simulink model "DDCU_wxt_v02"  (R2014a)
settings: Solver=ode45  StartTime=0.0  StopTime=50  FixedStep=0.0005  RelTol=1e-3
values from neighbouring files (symbols this model uses):
  ag_thr = 0.4*g    (= 3.924)    [Veh_Par_wxt.m]
  B = 2.25    [Veh_Par_wxt.m]
  bra_pre_em = 12    [Veh_Par_wxt.m]
  bra_pre_gz2 = 12/3    (= 4)    [Veh_Par_wxt.m]
  bra_pre_gz34 = 12/3    (= 4)    [Veh_Par_wxt.m]
  bra_pre_yd = 12/2    (= 6)    [Veh_Par_wxt.m]
  brakepre_dem_data = [0 1 2 3 4 5 6 7 8 9 10 11 12]    [Veh_Par_wxt.m]
  brakeTrq_dem_data = [0 218.198 436.396 654.594 872.792 1090.99 1309.188 1527.386 1745.584 1963.782 2181.98 2400.178 2618.376]    [Veh_Par_wxt.m]
  bratrq_max = 4*2618.376    (= 10473.504)    [Veh_Par_wxt.m]
  eff_tran = 0.75    [Veh_Par_wxt.m]
  G = Mass*g    (= 36297)    [Veh_Par_wxt.m]
  kd1 = 1    [Veh_Par_wxt.m]
  kd2 = 1    [Veh_Par_wxt.m]
  kd3 = 1    [Veh_Par_wxt.m]
  ki1 = 1    [Veh_Par_wxt.m]
  ki2 = 1    [Veh_Par_wxt.m]
  ki3 = 1    [Veh_Par_wxt.m]
  kp1 = 1    [Veh_Par_wxt.m]
  kp2 = 1    [Veh_Par_wxt.m]
  kp3 = 1    [Veh_Par_wxt.m]
  L = 3.12    [Veh_Par_wxt.m]
  Radius = 0.20    (= 0.2)    [Veh_Par_wxt.m]
  s_opt_yi_add = 0.05    [Veh_Par_wxt.m]
  s_opt_zhuan_add = 0.05    [Veh_Par_wxt.m]
  spd_map_mot = [0 100 200 300 360 400 500 600 700 800 900]*tras_ratio    [Veh_Par_wxt.m]
  speed_thr_park = 5/3.6/Radius*30/pi    (= 66.3145596216)    [Veh_Par_wxt.m]
  trq_map_mot = [1200 1200 1200 1200 1200 1080 864 720 617 540 480]/tras_ratio    [Veh_Par_wxt.m]
  v_thr1_b = 5    [Veh_Par_wxt.m]
  v_thr2_b = 20    [Veh_Par_wxt.m]
  v_thr_park = 5    [Veh_Par_wxt.m]
undefined symbols (not defined in the file or in its folder): DiscIntNeverNeededParam
libraries: simulink x17, Solver_SF x1
(part 1 of 5)
settings Model: Creator=wxt  LastModifiedBy=wxt

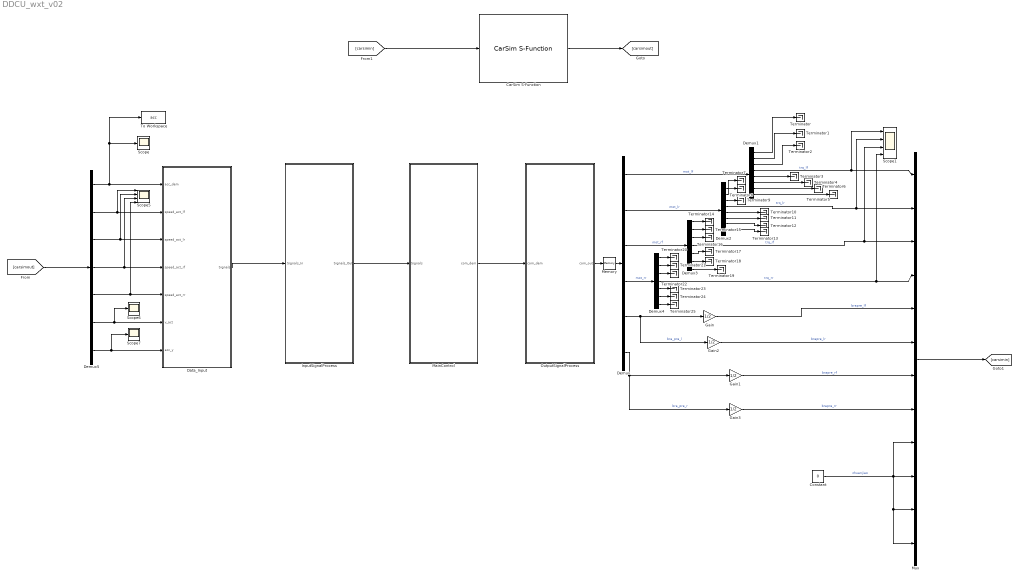
== system DDCU_wxt_v02 ==
  CarSim S-Function : Solver_SF/CarSim S-Function  Priority=1  VehicleCode=i_i  SIMFILE=lqddcuv01
  Constant : Constant  Value=0
  Data_Input : Subsystem
  Demux : Demux  Outputs=6
  Demux1 : Demux  Outputs=8
  Demux2 : Demux  Outputs=8
  Demux3 : Demux  Outputs=7
  Demux4 : Demux  Outputs=7
  Demux5 : Demux  Outputs=7
  Gain{,1..3} (4 alike) : Gain  Gain=1/2
  InputSignalProcess : Subsystem
  MainControl : Subsystem
  Memory : Memory
  Mux : Mux  Inputs=12
  OutputSignalProcess : Subsystem
  Scope : Scope
  Scope1 : Scope  NumInputPorts=4
      settings: YMin=-5~-5~-5~-5  YMax=5~5~5~5
  Scope5 : Scope  NumInputPorts=4
      settings: YMin=-5~-5~-5~-5  YMax=5~5~5~5  SaveName=ScopeData5
  Scope6 : Scope
      settings: SaveName=ScopeData6
  Scope7 : Scope
      settings: SaveName=ScopeData7
  Terminator{,1..25} (26 alike) : Terminator
  To Workspace : ToWorkspace  VariableName=acc  SampleTime=-1
  wires:
  Data_Input/1(Signals) -> InputSignalProcess/1(Signals_In)
  InputSignalProcess/1(Signals_Out) -> MainControl/1(Signals)
  MainControl/1(com_dem) -> OutputSignalProcess/1(com_dem)
  OutputSignalProcess/1(com_out) -> Memory/1
  Demux/1 -> Demux1/1  "mot_lf"
  Demux/2 -> Demux2/1  "mot_lr"
  Demux/3 -> Demux3/1  "mot_rf"
  Demux/4 -> Demux4/1  "mot_rr"
  Demux/5 -> Gain2/1, Gain/1  "bra_pre_l"
  Demux/6 -> Gain3/1, Gain1/1  "bra_pre_r"
  Demux1/4 -> Mux/1, Scope1/1  "trq_lf"
  Demux2/4 -> Mux/2, Scope1/2  "trq_lr"
  Demux3/4 -> Mux/3, Scope1/3  "trq_rf"
  Demux4/4 -> Mux/4, Scope1/4  "trq_rr"
  Gain/1 -> Mux/5  "brapre_lf"
  Gain1/1 -> Mux/7  "brapre_rf"
  Gain2/1 -> Mux/6  "brapre_lr"
  Gain3/1 -> Mux/8  "brapre_rr"
  Constant/1 -> Mux/9, Mux/10, Mux/12, Mux/11  "zhuanjiao"
  CarSim S-Function/1 -> [carsimout]
  [carsimout] -> Demux5/1
  Demux5/1 -> Data_Input/1(acc_dem), To Workspace/1, Scope/1
  Demux5/2 -> Scope5/1, Data_Input/2(speed_act_lf)
  Demux5/3 -> Data_Input/3(speed_act_lr), Scope5/2
  Demux5/4 -> Data_Input/4(speed_act_rf), Scope5/3
  Demux5/5 -> Data_Input/5(speed_act_rr), Scope5/4
  Demux5/6 -> Scope6/1, Data_Input/6(v_act)
  [carsimin] -> CarSim S-Function/1
  Mux/1 -> [carsimin]
  Demux5/7 -> Scope7/1, Data_Input/7(acc_y)
  Demux1/1 -> Terminator/1
  Demux1/2 -> Terminator1/1
  Demux1/3 -> Terminator2/1
  Demux1/5 -> Terminator3/1
  Demux1/6 -> Terminator4/1
  Demux1/7 -> Terminator5/1
  Demux1/8 -> Terminator6/1
  Demux2/3 -> Terminator9/1
  Demux2/2 -> Terminator8/1
  Demux2/1 -> Terminator7/1
  Demux2/5 -> Terminator10/1
  Demux2/6 -> Terminator11/1
  Demux2/7 -> Terminator12/1
  Demux2/8 -> Terminator13/1
  Demux3/1 -> Terminator14/1
  Demux3/2 -> Terminator15/1
  Demux3/3 -> Terminator16/1
  Demux3/5 -> Terminator17/1
  Demux3/6 -> Terminator18/1
  Demux3/7 -> Terminator19/1
  Demux4/1 -> Terminator20/1
  Demux4/2 -> Terminator21/1
  Demux4/3 -> Terminator22/1
  Demux4/5 -> Terminator23/1
  Demux4/6 -> Terminator24/1
  Demux4/7 -> Terminator25/1
  Memory/1 -> Demux/1

== system DDCU_wxt_v02/Data_Input ==
  acc_dem : Inport
  speed_act_lf : Inport  Port=2
  speed_act_lr : Inport  Port=3
  speed_act_rf : Inport  Port=4
  speed_act_rr : Inport  Port=5
  v_act : Inport  Port=6
  acc_y : Inport  Port=7
  BraSystem : Subsystem
  Bus Creator : BusCreator  Inputs=6
  Constant{,6..12} (8 alike) : Constant  Value=0
  Constant1 : Constant
  Constant2 : Constant  Value=1000
  Constant3 : Constant  Value=-1000
  Constant4 : Constant  Value=85
  Constant5 : Constant  Value=-85
  DriveMotor : Subsystem
  IMU : Subsystem
  Suspension : Subsystem
  Suspension1 : Subsystem
  YaoKong : Subsystem
  Signals : Outport
  wires:
  DriveMotor/1(DriveMotor) -> Bus Creator/2
  BraSystem/1(BraPre) -> Bus Creator/3
  YaoKong/1(YaoKong_dem) -> Bus Creator/1
  IMU/1(IMU) -> Bus Creator/4
  Suspension/1(Center_of_Mass) -> Bus Creator/5
  Bus Creator/1 -> Signals/1
  Suspension1/1(Bat) -> Bus Creator/6
  acc_dem/1 -> YaoKong/2(acc_dem)
  Constant/1 -> YaoKong/3(steer_dem), YaoKong/4(brake_dem), YaoKong/5(brake_emerg), YaoKong/6(HAC)
  Constant1/1 -> YaoKong/1(mode_dem)
  Constant2/1 -> DriveMotor/18(trqlimU_dig_rr), DriveMotor/13(trqlimU_dig_rf), DriveMotor/8(trqlimU_dig_lr), DriveMotor/3(trqlimU_dig_lf)
  Constant3/1 -> DriveMotor/4(trqlimL_dig_lf), DriveMotor/9(trqlimL_dig_lr), DriveMotor/14(trqlimL_dig_rf), DriveMotor/19(trqlimL_dig_rr)
  speed_act_lf/1 -> DriveMotor/1(speed_act_lf)
  speed_act_lr/1 -> DriveMotor/6(speed_act_lr)
  speed_act_rf/1 -> DriveMotor/11(speed_act_rf)
  speed_act_rr/1 -> DriveMotor/16(speed_act_rr)
  v_act/1 -> IMU/1(v_act)
  Constant4/1 -> Suspension1/1(pwr_dis_bat)
  Constant5/1 -> Suspension1/2(pwr_chg_bat)
  Constant6/1 -> BraSystem/1(BraPre_act_l)
  Constant7/1 -> BraSystem/2(BraPre_act_r)
  acc_y/1 -> IMU/9(acc_y)
  Constant8/1 -> DriveMotor/7(trq_act_lr), DriveMotor/12(trq_act_rf), DriveMotor/17(trq_act_rr), DriveMotor/2(trq_act_lf)
  Constant9/1 -> DriveMotor/20(guzhang_rr), DriveMotor/15(guzhang_rf), DriveMotor/10(guzhang_lr), DriveMotor/5(guzhang_lf)
  Constant10/1 -> IMU/3(dis_north), IMU/4(dis_sky), IMU/5(hangxiangangle), IMU/7(henggunangle), IMU/8(acc_x), IMU/6(fuyangangle), IMU/2(dis_east)
  Constant11/1 -> IMU/13(jiaosudu_z), IMU/12(jiaosudu_y), IMU/10(acc_z), IMU/11(jiaosudu_x)
  Constant12/1 -> Suspension/1(location_center)

== system DDCU_wxt_v02/InputSignalProcess ==
  note: 注：所有的单位转换都发生在此模块
      | 速度 km/h
      | 角速度 rpm
      | 加速度信号0-100
      | 制动信号0-100
      | 向左为正
  Signals_In : Inport
  Signals_Out : Outport
  wires:
  Signals_In/1 -> Signals_Out/1

== system DDCU_wxt_v02/MainControl ==
  Signals : Inport
  mode_control : Subsystem
  mode_switch : Subsystem
  com_dem : Outport
  wires:
  Signals/1 -> mode_control/2(Signals), mode_switch/1(Signals)
  mode_switch/1(mode_dem_out) -> mode_control/1(mode_dem_out)
  mode_control/1(com_dem) -> com_dem/1

== system DDCU_wxt_v02/OutputSignalProcess ==
  com_dem : Inport
  com_out : Outport
  wires:
  com_dem/1 -> com_out/1

== system DDCU_wxt_v02/Data_Input/BraSystem ==
  BraPre_act_l : Inport
  BraPre_act_r : Inport  Port=2
  Bus Creator : BusCreator  Inputs=2
  BraPre : Outport
  wires:
  BraPre_act_l/1 -> Bus Creator/1  "BraPre_act"
  Bus Creator/1 -> BraPre/1  "BraPre"
  BraPre_act_r/1 -> Bus Creator/2  "BraPre_act_r"

== system DDCU_wxt_v02/Data_Input/DriveMotor ==
  speed_act_lf : Inport
  trq_act_lf : Inport  Port=2
  trqlimU_dig_lf : Inport  Port=3
  trqlimL_dig_lf : Inport  Port=4
  guzhang_lf : Inport  Port=5
  speed_act_lr : Inport  Port=6
  trq_act_lr : Inport  Port=7
  trqlimU_dig_lr : Inport  Port=8
  trqlimL_dig_lr : Inport  Port=9
  guzhang_lr : Inport  Port=10
  speed_act_rf : Inport  Port=11
  trq_act_rf : Inport  Port=12
  trqlimU_dig_rf : Inport  Port=13
  trqlimL_dig_rf : Inport  Port=14
  guzhang_rf : Inport  Port=15
  speed_act_rr : Inport  Port=16
  trq_act_rr : Inport  Port=17
  trqlimU_dig_rr : Inport  Port=18
  trqlimL_dig_rr : Inport  Port=19
  guzhang_rr : Inport  Port=20
  Bus Creator : BusCreator  Inputs=20
  DriveMotor : Outport
  wires:
  Bus Creator/1 -> DriveMotor/1  "DriveMotor"
  trqlimL_dig_lr/1 -> Bus Creator/9  "trqlimL_dig_lr"
  trq_act_lf/1 -> Bus Creator/2  "trq_act_lf"
  trq_act_lr/1 -> Bus Creator/7  "trq_act_lr"
  trqlimL_dig_lf/1 -> Bus Creator/4  "trqlimL_dig_lf"
  trqlimU_dig_lf/1 -> Bus Creator/3  "trqlimU_dig_lf"
  trqlimU_dig_lr/1 -> Bus Creator/8  "trqlimU_dig_lr"
  speed_act_lf/1 -> Bus Creator/1  "speed_act_lf"
  speed_act_lr/1 -> Bus Creator/6  "speed_act_lr"
  guzhang_rf/1 -> Bus Creator/15  "guzhang_rf"
  guzhang_lf/1 -> Bus Creator/5  "guzhang_lf"
  guzhang_lr/1 -> Bus Creator/10  "guzhang_lr"
  speed_act_rf/1 -> Bus Creator/11  "speed_act_rf"
  guzhang_rr/1 -> Bus Creator/20  "guzhang_rr"
  trq_act_rf/1 -> Bus Creator/12  "trq_act_rf"
  speed_act_rr/1 -> Bus Creator/16  "speed_act_rr"
  trqlimL_dig_rf/1 -> Bus Creator/14  "trqlimL_dig_rf"
  trq_act_rr/1 -> Bus Creator/17  "trq_act_rr"
  trqlimL_dig_rr/1 -> Bus Creator/19  "trqlimL_dig_rr"
  trqlimU_dig_rf/1 -> Bus Creator/13  "trqlimU_dig_rf"
  trqlimU_dig_rr/1 -> Bus Creator/18  "trqlimU_dig_rr"

== system DDCU_wxt_v02/Data_Input/IMU ==
  v_act : Inport
  dis_east : Inport  Port=2
  dis_north : Inport  Port=3
  dis_sky : Inport  Port=4
  hangxiangangle : Inport  Port=5
  fuyangangle : Inport  Port=6
  henggunangle : Inport  Port=7
  acc_x : Inport  Port=8
  acc_y : Inport  Port=9
  acc_z : Inport  Port=10
  jiaosudu_x : Inport  Port=11
  jiaosudu_y : Inport  Port=12
  jiaosudu_z : Inport  Port=13
  Bus Creator : BusCreator  Inputs=13
  IMU : Outport
  wires:
  Bus Creator/1 -> IMU/1  "IMU"
  dis_east/1 -> Bus Creator/2  "dis_east"
  hangxiangangle/1 -> Bus Creator/5  "hangxiangangle"
  dis_north/1 -> Bus Creator/3  "dis_north"
  dis_sky/1 -> Bus Creator/4  "dis_sky"
  fuyangangle/1 -> Bus Creator/6  "fuyangangle"
  acc_y/1 -> Bus Creator/9  "acc_y"
  henggunangle/1 -> Bus Creator/7  "henggunangle"
  acc_x/1 -> Bus Creator/8  "acc_x"
  acc_z/1 -> Bus Creator/10  "acc_z"
  jiaosudu_z/1 -> Bus Creator/13  "jiaosudu_z"
  jiaosudu_x/1 -> Bus Creator/11  "jiaosudu_x"
  jiaosudu_y/1 -> Bus Creator/12  "jiaosudu_y"
  v_act/1 -> Bus Creator/1  "v_act"

== system DDCU_wxt_v02/Data_Input/Suspension ==
  location_center : Inport
  Bus Creator : BusCreator  Inputs=1
  Center_of_Mass : Outport
  wires:
  Bus Creator/1 -> Center_of_Mass/1  "Center_of_Mass"
  location_center/1 -> Bus Creator/1  "location_center"

== system DDCU_wxt_v02/Data_Input/Suspension1 ==
  pwr_dis_bat : Inport
  pwr_chg_bat : Inport  Port=2
  Bus Creator : BusCreator  Inputs=2
  Bat : Outport
  wires:
  pwr_dis_bat/1 -> Bus Creator/1  "pwr_dis_bat"
  Bus Creator/1 -> Bat/1  "Bat"
  pwr_chg_bat/1 -> Bus Creator/2  "pwr_chg_bat"

== system DDCU_wxt_v02/Data_Input/YaoKong ==
  note: 上坡辅助系统(Hill-start Assist Control，HAC)
  mode_dem : Inport
  acc_dem : Inport  Port=2
  steer_dem : Inport  Port=3
  brake_dem : Inport  Port=4
  brake_emerg : Inport  Port=5
  HAC : Inport  Port=6
  Bus Creator : BusCreator  Inputs=6
  YaoKong_dem : Outport
  wires:
  steer_dem/1 -> Bus Creator/3  "steer_dem"
  acc_dem/1 -> Bus Creator/2  "acc_dem"
  brake_dem/1 -> Bus Creator/4  "brake_dem"
  mode_dem/1 -> Bus Creator/1  "mode_dem"
  Bus Creator/1 -> YaoKong_dem/1  "YaoKong"
  brake_emerg/1 -> Bus Creator/5  "brake_emerg"
  HAC/1 -> Bus Creator/6  "HAC"

== system DDCU_wxt_v02/MainControl/mode_control ==
  mode_dem_out : Inport
  Signals : Inport  Port=2
  Multiport Switch : MultiPortSwitch  DataPortOrder=Zero-based contiguous  Inputs=6
  Park : Subsystem  TreatAsAtomicUnit=on
  Switch Case : SwitchCase  CaseConditions={0,1,2,3,4,5}  ShowDefaultCase=off
  backward : Subsystem  Commented=on  TreatAsAtomicUnit=on
  center_steer : Subsystem  TreatAsAtomicUnit=on
  emergency_stop : Subsystem  TreatAsAtomicUnit=on
  forward : Subsystem  TreatAsAtomicUnit=on
  neutral : Subsystem  TreatAsAtomicUnit=on
  com_dem : Outport
  wires:
  mode_dem_out/1 -> Multiport Switch/1, Switch Case/1
  Signals/1 -> emergency_stop/1(Signals), center_steer/1(Signals), backward/1(Signals), neutral/1(Signals), forward/1(Signals), Park/1(Signals)
  Switch Case/1 -> Park/Action
  Switch Case/6 -> emergency_stop/Action
  Switch Case/5 -> center_steer/Action
  Switch Case/4 -> backward/Action
  Switch Case/3 -> neutral/Action
  Switch Case/2 -> forward/Action
  Park/1(park_dem) -> Multiport Switch/2
  forward/1(forward_dem) -> Multiport Switch/3
  backward/1(backward_dem) -> Multiport Switch/5
  neutral/1(neutral_dem) -> Multiport Switch/4
  center_steer/1(center_steer_dem) -> Multiport Switch/6
  emergency_stop/1(emergency_stop_dem) -> Multiport Switch/7
  Multiport Switch/1 -> com_dem/1

== system DDCU_wxt_v02/MainControl/mode_switch ==
  Signals : Inport
  Bus Selector : BusSelector  OutputSignals=YaoKong.mode_dem,YaoKong.brake_emerg,DriveMotor.speed_act_lf,DriveMotor.speed_act_lr,DriveMotor.speed_act_rf,DriveMotor.speed_act_rr,IMU.v_act
  Constant : Constant
  Constant1 : Constant  Value=v_thr_park
  Constant2 : Constant  Value=speed_thr_park
  Memory : Memory
  mode_switch : MATLAB Function  TreatAsAtomicUnit=on
  mode_dem_out : Outport
  wires:
  Memory/1 -> mode_switch/10(mode_dem_out_pre)
  Signals/1 -> Bus Selector/1
  Bus Selector/3 -> mode_switch/3(speed_act_lf)  "<speed_act_lf>"
  Bus Selector/2 -> mode_switch/2(brake_emerg)  "<brake_emerg>"
  Bus Selector/1 -> mode_switch/1(mode_dem)  "<mode_dem>"
  Bus Selector/5 -> mode_switch/5(speed_act_rf)  "<speed_act_rf>"
  Bus Selector/4 -> mode_switch/4(speed_act_lr)  "<speed_act_lr>"
  Bus Selector/6 -> mode_switch/6(speed_act_rr)  "<speed_act_rr>"
  Bus Selector/7 -> mode_switch/7(v_act)  "<v_act>"
  mode_switch/1(mode_dem_out) -> Memory/1
  Constant/1 -> mode_dem_out/1
  Constant2/1 -> mode_switch/9(speed_thr_park)
  Constant1/1 -> mode_switch/8(v_thr_park)

== system DDCU_wxt_v02/MainControl/mode_control/Park ==
  Signals : Inport
  Action Port : ActionPort  ActionType=case
  Mux : Mux  Inputs=6
  park : Subsystem
  park_dem : Outport
  wires:
  Signals/1 -> park/1(Signals)
  park/4(mot_rr) -> Mux/4
  park/3(mot_rf) -> Mux/3
  park/5(bra_pre_l) -> Mux/5
  park/2(mot_lr) -> Mux/2
  park/6(bra_pre_r) -> Mux/6
  park/1(mot_lf) -> Mux/1
  Mux/1 -> park_dem/1

== system DDCU_wxt_v02/MainControl/mode_control/backward ==
  Signals : Inport
  Action Port : ActionPort  ActionType=case
  Mux : Mux  Inputs=6
  backward : Subsystem
  backward_dem : Outport
  wires:
  Signals/1 -> backward/1(Signals)
  backward/4(mot_lr2) -> Mux/4
  backward/3(mot_lr1) -> Mux/3
  backward/5(bra_pre_l) -> Mux/5
  backward/2(mot_lr) -> Mux/2
  backward/6(bra_pre_r) -> Mux/6
  backward/1(mot_lf) -> Mux/1
  Mux/1 -> backward_dem/1

== system DDCU_wxt_v02/MainControl/mode_control/center_steer ==
  Signals : Inport
  Action Port : ActionPort  ActionType=case
  Mux : Mux  Inputs=6
  center_steer : Subsystem
  center_steer_dem : Outport
  wires:
  Mux/1 -> center_steer_dem/1
  center_steer/6(bra_pre_r) -> Mux/6
  center_steer/5(bra_pre_l) -> Mux/5
  Signals/1 -> center_steer/1(Signals)
  center_steer/1(mot_lf) -> Mux/1
  center_steer/2(mot_lr) -> Mux/2
  center_steer/4(mot_rr) -> Mux/4
  center_steer/3(mot_rf) -> Mux/3

== system DDCU_wxt_v02/MainControl/mode_control/emergency_stop ==
  Signals : Inport
  Action Port : ActionPort  ActionType=case
  Mux : Mux  Inputs=6
  emergency_stop : Subsystem
  emergency_stop_dem : Outport
  wires:
  Mux/1 -> emergency_stop_dem/1
  emergency_stop/1(mot_lf) -> Mux/1
  emergency_stop/6(bra_pre_r) -> Mux/6
  emergency_stop/4(mot_rr) -> Mux/4
  emergency_stop/5(bra_pre_l) -> Mux/5
  emergency_stop/3(mot_rf) -> Mux/3
  emergency_stop/2(mot_lr) -> Mux/2
  Signals/1 -> emergency_stop/1(Signals)

== system DDCU_wxt_v02/MainControl/mode_control/forward ==
  Signals : Inport
  Action Port : ActionPort  ActionType=case
  forward : Subsystem
  forward_dem : Outport
  wires:
  forward/1(forward_dem) -> forward_dem/1
  Signals/1 -> forward/1(Signals)

== system DDCU_wxt_v02/MainControl/mode_control/neutral ==
  Signals : Inport
  Action Port : ActionPort  ActionType=case
  Mux : Mux  Inputs=6
  neutral : Subsystem
  neutral_dem : Outport
  wires:
  Mux/1 -> neutral_dem/1
  Signals/1 -> neutral/1(Signals)
  neutral/2(mot_lr) -> Mux/2
  neutral/3(mot_rf) -> Mux/3
  neutral/1(mot_lf) -> Mux/1
  neutral/6(bra_pre_r) -> Mux/6
  neutral/5(bra_pre_l) -> Mux/5
  neutral/4(mot_rr) -> Mux/4

== system DDCU_wxt_v02/MainControl/mode_control/Park/park ==
  Signals : Inport
  1-D Lookup Table : Lookup_n-D  NumberOfTableDimensions=1  BreakpointsForDimension1=brakeTrq_dem_data  Table=brakepre_dem_data  InternalRulePriority=Speed  RndMeth=Simplest  InputSameDT=on
  1-D Lookup Table1 : Lookup_n-D  NumberOfTableDimensions=1  BreakpointsForDimension1=brakeTrq_dem_data  Table=brakepre_dem_data  InternalRulePriority=Speed  RndMeth=Simplest  InputSameDT=on
  Bus Selector : BusSelector  OutputSignals=YaoKong.brake_dem
  Constant : Constant  Value=bratrq_max
  Gain : Gain  Gain=1/2
  Gain1 : Gain  Gain=1/100
  Gain2 : Gain  Gain=1/2
  Gain3 : Gain  Gain=1/2
  HeartBeat : MATLAB Function  TreatAsAtomicUnit=on
  HeartBeat1 : MATLAB Function  TreatAsAtomicUnit=on
  Memory : Memory
  Memory1 : Memory
  Mux : Mux  Inputs=8
  Mux1 : Mux  Inputs=8
  Mux2 : Mux  Inputs=7
  Mux3 : Mux  Inputs=7
  Product : Product
  SpdLim_dem{,1..3} (4 alike) : Constant
  SpdSet_dem{,1..3} (4 alike) : Constant
  TrqLim_dem{,1..3} (4 alike) : Constant
  TrqSet_dem{,1..3} (4 alike) : Constant
  mot_drive{,1..3} (4 alike) : Constant
  mot_enable{,1..3} (4 alike) : Constant
  mot_mode{,1..3} (4 alike) : Constant
  mot_lf : Outport
  mot_lr : Outport  Port=2
  mot_rf : Outport  Port=3
  mot_rr : Outport  Port=4
  bra_pre_l : Outport  Port=5
  bra_pre_r : Outport  Port=6
  wires:
  mot_drive/1 -> Mux/3
  mot_mode/1 -> Mux/2
  TrqSet_dem/1 -> Mux/4
  mot_enable/1 -> Mux/1
  SpdSet_dem/1 -> Mux/5
  Mux/1 -> mot_lf/1
  Signals/1 -> Bus Selector/1
  1-D Lookup Table/1 -> bra_pre_l/1
  TrqLim_dem/1 -> Mux/6
  HeartBeat/1(life) -> Mux/8, Memory/1
  Memory/1 -> HeartBeat/1(life_pre)
  SpdLim_dem/1 -> Mux/7
  mot_drive1/1 -> Mux2/3
  mot_mode2/1 -> Mux2/2
  TrqSet_dem1/1 -> Mux2/4
  mot_enable2/1 -> Mux2/1
  SpdSet_dem1/1 -> Mux2/5
  Mux2/1 -> mot_rf/1
  TrqLim_dem1/1 -> Mux2/6
  SpdLim_dem1/1 -> Mux2/7
  mot_drive2/1 -> Mux1/3
  mot_mode1/1 -> Mux1/2
  TrqSet_dem2/1 -> Mux1/4
  mot_enable1/1 -> Mux1/1
  SpdSet_dem2/1 -> Mux1/5
  Mux1/1 -> mot_lr/1
  TrqLim_dem2/1 -> Mux1/6
  HeartBeat1/1(life) -> Mux1/8, Memory1/1
  Memory1/1 -> HeartBeat1/1(life_pre)
  SpdLim_dem2/1 -> Mux1/7
  mot_drive3/1 -> Mux3/3
  mot_mode3/1 -> Mux3/2
  TrqSet_dem3/1 -> Mux3/4
  mot_enable3/1 -> Mux3/1
  SpdSet_dem3/1 -> Mux3/5
  Mux3/1 -> mot_rr/1
  TrqLim_dem3/1 -> Mux3/6
  SpdLim_dem3/1 -> Mux3/7
  Constant/1 -> Product/1
  Bus Selector/1 -> Gain1/1  "<brake_dem>"
  Product/1 -> Gain/1
  Gain/1 -> Gain3/1, Gain2/1
  Gain1/1 -> Product/2
  Gain2/1 -> 1-D Lookup Table/1
  Gain3/1 -> 1-D Lookup Table1/1
  1-D Lookup Table1/1 -> bra_pre_r/1

== system DDCU_wxt_v02/MainControl/mode_control/backward/backward ==
  Signals : Inport
  Bus Selector : BusSelector  OutputSignals=YaoKong.brake_dem
  Gain : Gain  Gain=1/2
  Mux{,1..3} (4 alike) : Mux  Inputs=5
  Spd_dem{,1..3} (4 alike) : Constant
  Trq_dem{,1..3} (4 alike) : Constant
  mot_enable{,1..3} (4 alike) : Constant
  mot_mode{,1..3} (4 alike) : Constant
  mot_move{,1..3} (4 alike) : Constant
  mot_lf : Outport
  mot_lr : Outport  Port=2
  mot_lr1 : Outport  Port=3
  mot_lr2 : Outport  Port=4
  bra_pre_l : Outport  Port=5
  bra_pre_r : Outport  Port=6
  wires:
  mot_move/1 -> Mux/3
  mot_mode/1 -> Mux/2
  Trq_dem/1 -> Mux/4
  mot_enable/1 -> Mux/1
  Spd_dem/1 -> Mux/5
  Mux/1 -> mot_lf/1
  mot_move1/1 -> Mux1/3
  mot_mode1/1 -> Mux1/2
  Trq_dem1/1 -> Mux1/4
  mot_enable1/1 -> Mux1/1
  Spd_dem1/1 -> Mux1/5
  Mux1/1 -> mot_lr/1
  mot_move2/1 -> Mux2/3
  mot_mode2/1 -> Mux2/2
  Trq_dem2/1 -> Mux2/4
  mot_enable2/1 -> Mux2/1
  Spd_dem2/1 -> Mux2/5
  Mux2/1 -> mot_lr1/1
  mot_move3/1 -> Mux3/3
  mot_mode3/1 -> Mux3/2
  Trq_dem3/1 -> Mux3/4
  mot_enable3/1 -> Mux3/1
  Spd_dem3/1 -> Mux3/5
  Mux3/1 -> mot_lr2/1
  Signals/1 -> Bus Selector/1
  Bus Selector/1 -> Gain/1  "<brake_dem>"
  Gain/1 -> bra_pre_r/1, bra_pre_l/1

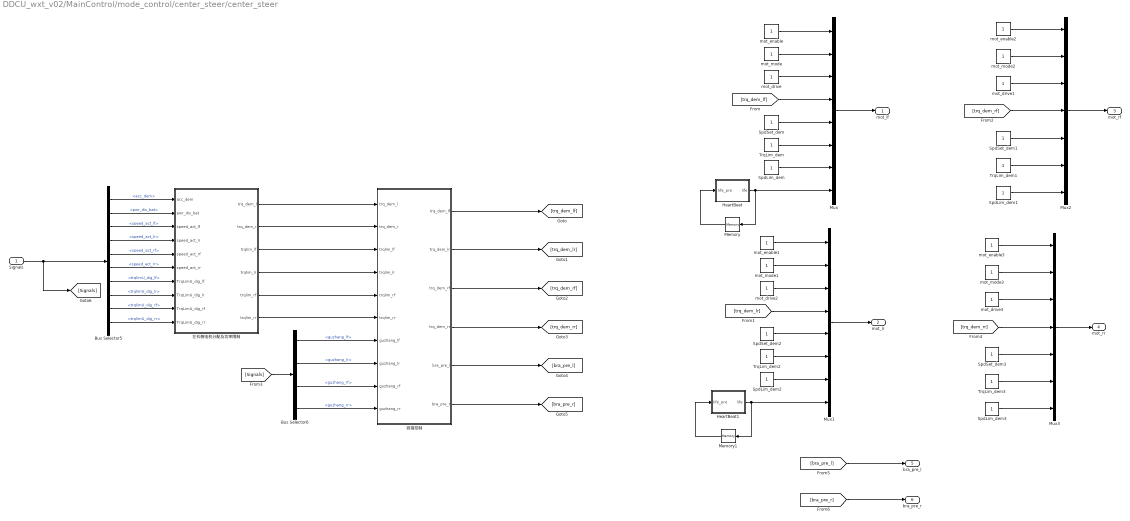
== system DDCU_wxt_v02/MainControl/mode_control/center_steer/center_steer ==
  Signals : Inport
  Bus Selector5 : BusSelector  OutputSignals=YaoKong.acc_dem,Bat.pwr_dis_bat,DriveMotor.speed_act_lf,DriveMotor.speed_act_lr,DriveMotor.speed_act_rf,DriveMotor.speed_act_rr,DriveMotor.trqlimU_dig_lf,DriveMotor.trqlimU_dig_lr,DriveMotor.trqlimU_dig_rf,DriveMotor.trqlimU_dig_rr
  Bus Selector6 : BusSelector  OutputSignals=DriveMotor.guzhang_lf,DriveMotor.guzhang_lr,DriveMotor.guzhang_rf,DriveMotor.guzhang_rr
  HeartBeat : MATLAB Function  TreatAsAtomicUnit=on
  HeartBeat1 : MATLAB Function  TreatAsAtomicUnit=on
  Memory : Memory
  Memory1 : Memory
  Mux : Mux  Inputs=8
  Mux1 : Mux  Inputs=8
  Mux2 : Mux  Inputs=7
  Mux3 : Mux  Inputs=7
  SpdLim_dem{,1..3} (4 alike) : Constant
  SpdSet_dem{,1..3} (4 alike) : Constant
  TrqLim_dem{,1..3} (4 alike) : Constant
  mot_drive{,1..3} (4 alike) : Constant
  mot_enable{,1..3} (4 alike) : Constant
  mot_mode{,1..3} (4 alike) : Constant
  容错控制 : Subsystem
  左右侧电机分配及功率限制 : Subsystem
  mot_lf : Outport
  mot_lr : Outport  Port=2
  mot_rf : Outport  Port=3
  mot_rr : Outport  Port=4
  bra_pre_l : Outport  Port=5
  bra_pre_r : Outport  Port=6
  wires:
  Signals/1 -> [Signals], Bus Selector5/1
  Bus Selector5/2 -> 左右侧电机分配及功率限制/2(pwr_dis_bat)  "<pwr_dis_bat>"
  Bus Selector5/3 -> 左右侧电机分配及功率限制/3(speed_act_lf)  "<speed_act_lf>"
  Bus Selector5/4 -> 左右侧电机分配及功率限制/4(speed_act_lr)  "<speed_act_lr>"
  Bus Selector5/5 -> 左右侧电机分配及功率限制/5(speed_act_rf)  "<speed_act_rf>"
  Bus Selector5/6 -> 左右侧电机分配及功率限制/6(speed_act_rr)  "<speed_act_rr>"
  Bus Selector5/10 -> 左右侧电机分配及功率限制/10(TrqLimU_dig_rr)  "<trqlimU_dig_rr>"
  Bus Selector5/9 -> 左右侧电机分配及功率限制/9(TrqLimU_dig_rf)  "<trqlimU_dig_rf>"
  Bus Selector5/7 -> 左右侧电机分配及功率限制/7(TrqLimU_dig_lf)  "<trqlimU_dig_lf>"
  Bus Selector5/8 -> 左右侧电机分配及功率限制/8(TrqLimU_dig_lr)  "<trqlimU_dig_lr>"
  [Signals] -> Bus Selector6/1
  左右侧电机分配及功率限制/2(trq_dem_r) -> 容错控制/2(trq_dem_r)
  左右侧电机分配及功率限制/1(trq_dem_l) -> 容错控制/1(trq_dem_l)
  Bus Selector6/4 -> 容错控制/10(guzhang_rr)  "<guzhang_rr>"
  Bus Selector6/3 -> 容错控制/9(guzhang_rf)  "<guzhang_rf>"
  Bus Selector6/2 -> 容错控制/8(guzhang_lr)  "<guzhang_lr>"
  Bus Selector6/1 -> 容错控制/7(guzhang_lf)  "<guzhang_lf>"
  左右侧电机分配及功率限制/5(trqlim_rf) -> 容错控制/5(trqlim_rf)
  左右侧电机分配及功率限制/4(trqlim_lr) -> 容错控制/4(trqlim_lr)
  左右侧电机分配及功率限制/6(trqlim_rr) -> 容错控制/6(trqlim_rr)
  左右侧电机分配及功率限制/3(trqlim_lf) -> 容错控制/3(trqlim_lf)
  Bus Selector5/1 -> 左右侧电机分配及功率限制/1(acc_dem)  "<acc_dem>"
  容错控制/1(trq_dem_lf) -> [trq_dem_lf]
  容错控制/3(trq_dem_rf) -> [trq_dem_rf]
  容错控制/4(trq_dem_rr) -> [trq_dem_rr]
  容错控制/5(bra_pre_l) -> [bra_pre_l]
  容错控制/6(bra_pre_r) -> [bra_pre_r]
  容错控制/2(trq_dem_lr) -> [trq_dem_lr]
  mot_drive/1 -> Mux/3
  mot_mode/1 -> Mux/2
  [trq_dem_lf] -> Mux/4
  mot_enable/1 -> Mux/1
  SpdSet_dem/1 -> Mux/5
  Mux/1 -> mot_lf/1
  TrqLim_dem/1 -> Mux/6
  HeartBeat/1(life) -> Mux/8, Memory/1
  Memory/1 -> HeartBeat/1(life_pre)
  SpdLim_dem/1 -> Mux/7
  mot_drive1/1 -> Mux2/3
  mot_mode2/1 -> Mux2/2
  [trq_dem_rf] -> Mux2/4
  mot_enable2/1 -> Mux2/1
  SpdSet_dem1/1 -> Mux2/5
  Mux2/1 -> mot_rf/1
  TrqLim_dem1/1 -> Mux2/6
  SpdLim_dem1/1 -> Mux2/7
  mot_drive2/1 -> Mux1/3
  mot_mode1/1 -> Mux1/2
  [trq_dem_lr] -> Mux1/4
  mot_enable1/1 -> Mux1/1
  SpdSet_dem2/1 -> Mux1/5
  Mux1/1 -> mot_lr/1
  TrqLim_dem2/1 -> Mux1/6
  HeartBeat1/1(life) -> Mux1/8, Memory1/1
  Memory1/1 -> HeartBeat1/1(life_pre)
  SpdLim_dem2/1 -> Mux1/7
  mot_drive3/1 -> Mux3/3
  mot_mode3/1 -> Mux3/2
  [trq_dem_rr] -> Mux3/4
  mot_enable3/1 -> Mux3/1
  SpdSet_dem3/1 -> Mux3/5
  Mux3/1 -> mot_rr/1
  TrqLim_dem3/1 -> Mux3/6
  SpdLim_dem3/1 -> Mux3/7
  [bra_pre_l] -> bra_pre_l/1
  [bra_pre_r] -> bra_pre_r/1

== system DDCU_wxt_v02/MainControl/mode_control/emergency_stop/emergency_stop ==
  Signals : Inport
  Bus Selector : BusSelector  OutputSignals=YaoKong.brake_dem
  Constant : Constant  Value=bra_pre_em
  HeartBeat : MATLAB Function  TreatAsAtomicUnit=on
  HeartBeat1 : MATLAB Function  TreatAsAtomicUnit=on
  Memory : Memory
  Memory1 : Memory
  Mux : Mux  Inputs=8
  Mux1 : Mux  Inputs=8
  Mux2 : Mux  Inputs=7
  Mux3 : Mux  Inputs=7
  SpdLim_dem{,1..3} (4 alike) : Constant
  SpdSet_dem{,1..3} (4 alike) : Constant
  Terminator : Terminator
  TrqLim_dem{,1..3} (4 alike) : Constant
  TrqSet_dem{,1..3} (4 alike) : Constant
  mot_drive{,1..3} (4 alike) : Constant
  mot_enable{,1..3} (4 alike) : Constant
  mot_mode{,1..3} (4 alike) : Constant
  mot_lf : Outport
  mot_lr : Outport  Port=2
  mot_rf : Outport  Port=3
  mot_rr : Outport  Port=4
  bra_pre_l : Outport  Port=5
  bra_pre_r : Outport  Port=6
  wires:
  mot_drive/1 -> Mux/3
  mot_mode/1 -> Mux/2
  TrqSet_dem/1 -> Mux/4
  mot_enable/1 -> Mux/1
  SpdSet_dem/1 -> Mux/5
  Mux/1 -> mot_lf/1
  Signals/1 -> Bus Selector/1
  Bus Selector/1 -> Terminator/1  "<brake_dem>"
  TrqLim_dem/1 -> Mux/6
  HeartBeat/1(life) -> Mux/8, Memory/1
  Memory/1 -> HeartBeat/1(life_pre)
  SpdLim_dem/1 -> Mux/7
  mot_drive1/1 -> Mux2/3
  mot_mode2/1 -> Mux2/2
  TrqSet_dem1/1 -> Mux2/4
  mot_enable2/1 -> Mux2/1
  SpdSet_dem1/1 -> Mux2/5
  Mux2/1 -> mot_rf/1
  TrqLim_dem1/1 -> Mux2/6
  SpdLim_dem1/1 -> Mux2/7
  mot_drive2/1 -> Mux1/3
  mot_mode1/1 -> Mux1/2
  TrqSet_dem2/1 -> Mux1/4
  mot_enable1/1 -> Mux1/1
  SpdSet_dem2/1 -> Mux1/5
  Mux1/1 -> mot_lr/1
  TrqLim_dem2/1 -> Mux1/6
  HeartBeat1/1(life) -> Mux1/8, Memory1/1
  Memory1/1 -> HeartBeat1/1(life_pre)
  SpdLim_dem2/1 -> Mux1/7
  mot_drive3/1 -> Mux3/3
  mot_mode3/1 -> Mux3/2
  TrqSet_dem3/1 -> Mux3/4
  mot_enable3/1 -> Mux3/1
  SpdSet_dem3/1 -> Mux3/5
  Mux3/1 -> mot_rr/1
  TrqLim_dem3/1 -> Mux3/6
  SpdLim_dem3/1 -> Mux3/7
  Constant/1 -> bra_pre_r/1, bra_pre_l/1

== system DDCU_wxt_v02/MainControl/mode_control/forward/forward ==
  Signals : Inport
  Brake : Subsystem  TreatAsAtomicUnit=on
  Bus Selector : BusSelector  OutputSignals=YaoKong.acc_dem
  Constant : Constant  Value=0.15
  Drive : Subsystem  TreatAsAtomicUnit=on
  MATLAB Function : MATLAB Function  TreatAsAtomicUnit=on
  Multiport Switch : MultiPortSwitch  DataPortOrder=Zero-based contiguous  Inputs=2
  Switch Case1 : SwitchCase  CaseConditions={0,1}  ShowDefaultCase=off
  forward_dem : Outport
  wires:
  Signals/1 -> Brake/1(Signals), Drive/1(Signals), Bus Selector/1
  Multiport Switch/1 -> forward_dem/1
  Switch Case1/1 -> Drive/Action
  Switch Case1/2 -> Brake/Action
  Bus Selector/1 -> MATLAB Function/1(acc_dem)  "<acc_dem>"
  MATLAB Function/1(y) -> Multiport Switch/1, Switch Case1/1
  Drive/1(forward_dem) -> Multiport Switch/2
  Brake/1(forward_dem) -> Multiport Switch/3
  Constant/1 -> Brake/2(s_opt_yi)

== system DDCU_wxt_v02/MainControl/mode_control/neutral/neutral ==
  Signals : Inport
  Bus Selector : BusSelector  OutputSignals=YaoKong.brake_dem
  Constant : Constant  Value=0
  Gain : Gain  Gain=1/2
  HeartBeat : MATLAB Function  TreatAsAtomicUnit=on
  HeartBeat1 : MATLAB Function  TreatAsAtomicUnit=on
  Memory : Memory
  Memory1 : Memory
  Mux : Mux  Inputs=8
  Mux1 : Mux  Inputs=8
  Mux2 : Mux  Inputs=7
  Mux3 : Mux  Inputs=7
  SpdLim_dem{,1..3} (4 alike) : Constant
  SpdSet_dem{,1..3} (4 alike) : Constant
  Terminator : Terminator
  TrqLim_dem{,1..3} (4 alike) : Constant
  TrqSet_dem{,1..3} (4 alike) : Constant
  mot_drive{,1..3} (4 alike) : Constant
  mot_enable{,1..3} (4 alike) : Constant
  mot_mode{,1..3} (4 alike) : Constant
  mot_lf : Outport
  mot_lr : Outport  Port=2
  mot_rf : Outport  Port=3
  mot_rr : Outport  Port=4
  bra_pre_l : Outport  Port=5
  bra_pre_r : Outport  Port=6
  wires:
  mot_drive/1 -> Mux/3
  mot_mode/1 -> Mux/2
  TrqSet_dem/1 -> Mux/4
  mot_enable/1 -> Mux/1
  SpdSet_dem/1 -> Mux/5
  Mux/1 -> mot_lf/1
  Signals/1 -> Bus Selector/1
  Bus Selector/1 -> Gain/1  "<brake_dem>"
  TrqLim_dem/1 -> Mux/6
  HeartBeat/1(life) -> Mux/8, Memory/1
  Memory/1 -> HeartBeat/1(life_pre)
  SpdLim_dem/1 -> Mux/7
  mot_drive1/1 -> Mux2/3
  mot_mode2/1 -> Mux2/2
  TrqSet_dem1/1 -> Mux2/4
  mot_enable2/1 -> Mux2/1
  SpdSet_dem1/1 -> Mux2/5
  Mux2/1 -> mot_rf/1
  TrqLim_dem1/1 -> Mux2/6
  SpdLim_dem1/1 -> Mux2/7
  mot_drive2/1 -> Mux1/3
  mot_mode1/1 -> Mux1/2
  TrqSet_dem2/1 -> Mux1/4
  mot_enable1/1 -> Mux1/1
  SpdSet_dem2/1 -> Mux1/5
  Mux1/1 -> mot_lr/1
  TrqLim_dem2/1 -> Mux1/6
  HeartBeat1/1(life) -> Mux1/8, Memory1/1
  Memory1/1 -> HeartBeat1/1(life_pre)
  SpdLim_dem2/1 -> Mux1/7
  mot_drive3/1 -> Mux3/3
  mot_mode3/1 -> Mux3/2
  TrqSet_dem3/1 -> Mux3/4
  mot_enable3/1 -> Mux3/1
  SpdSet_dem3/1 -> Mux3/5
  Mux3/1 -> mot_rr/1
  TrqLim_dem3/1 -> Mux3/6
  SpdLim_dem3/1 -> Mux3/7
  Gain/1 -> Terminator/1
  Constant/1 -> bra_pre_r/1, bra_pre_l/1

== system DDCU_wxt_v02/MainControl/mode_control/center_steer/center_steer/容错控制 ==
  trq_dem_l : Inport
  trq_dem_r : Inport  Port=2
  trqlim_lf : Inport  Port=3
  trqlim_lr : Inport  Port=4
  trqlim_rf : Inport  Port=5
  trqlim_rr : Inport  Port=6
  guzhang_lf : Inport  Port=7
  guzhang_lr : Inport  Port=8
  guzhang_rf : Inport  Port=9
  guzhang_rr : Inport  Port=10
  Constant : Constant  Value=bra_pre_yd
  MATLAB Function : MATLAB Function  TreatAsAtomicUnit=on
  trq_dem_lf : Outport
  trq_dem_lr : Outport  Port=2
  trq_dem_rf : Outport  Port=3
  trq_dem_rr : Outport  Port=4
  bra_pre_l : Outport  Port=5
  bra_pre_r : Outport  Port=6
  wires:
  guzhang_lr/1 -> MATLAB Function/8(guzhang_lr)
  guzhang_rf/1 -> MATLAB Function/9(guzhang_rf)
  guzhang_rr/1 -> MATLAB Function/10(guzhang_rr)
  guzhang_lf/1 -> MATLAB Function/7(guzhang_lf)
  trq_dem_r/1 -> MATLAB Function/2(trq_dem_r)
  trqlim_lr/1 -> MATLAB Function/4(trqlim_lr)
  trq_dem_l/1 -> MATLAB Function/1(trq_dem_l)
  trqlim_rf/1 -> MATLAB Function/5(trqlim_rf)
  trqlim_rr/1 -> MATLAB Function/6(trqlim_rr)
  trqlim_lf/1 -> MATLAB Function/3(trqlim_lf)
  MATLAB Function/1(trq_dem_lf) -> trq_dem_lf/1
  MATLAB Function/2(trq_dem_lr) -> trq_dem_lr/1
  MATLAB Function/3(trq_dem_rf) -> trq_dem_rf/1
  MATLAB Function/4(trq_dem_rr) -> trq_dem_rr/1
  MATLAB Function/5(bra_pre_l) -> bra_pre_l/1
  MATLAB Function/6(bra_pre_r) -> bra_pre_r/1
  Constant/1 -> MATLAB Function/11(bra_pre_yd)

== system DDCU_wxt_v02/MainControl/mode_control/center_steer/center_steer/左右侧电机分配及功率限制 ==
  acc_dem : Inport
  pwr_dis_bat : Inport  Port=2
  speed_act_lf : Inport  Port=3
  speed_act_lr : Inport  Port=4
  speed_act_rf : Inport  Port=5
  speed_act_rr : Inport  Port=6
  TrqLimU_dig_lf : Inport  Port=7
  TrqLimU_dig_lr : Inport  Port=8
  TrqLimU_dig_rf : Inport  Port=9
  TrqLimU_dig_rr : Inport  Port=10
  Add1 : Sum  Inputs=++++
  Add3 : Sum  Inputs=++++
  Constant : Constant  Value=9549
  Divide : Product  Inputs=**/
  Gain : Gain  Gain=1/4
  Gain1 : Gain  Gain=1/2
  MinMax{,3..6} (5 alike) : MinMax  Inputs=2
  Product : Product
  mot_map{,1..3} (4 alike) : Lookup_n-D  NumberOfTableDimensions=1  BreakpointsForDimension1=spd_map_mot  Table=trq_map_mot  InternalRulePriority=Speed  RndMeth=Simplest  InputSameDT=on
  trq_dem_l : Outport
  trq_dem_r : Outport  Port=2
  trqlim_lf : Outport  Port=3
  trqlim_lr : Outport  Port=4
  trqlim_rf : Outport  Port=5
  trqlim_rr : Outport  Port=6
  wires:
  speed_act_rf/1 -> mot_map2/1, Add1/3
  speed_act_lr/1 -> mot_map1/1, Add1/2
  speed_act_rr/1 -> mot_map3/1, Add1/4
  speed_act_lf/1 -> mot_map/1, Add1/1
  Add1/1 -> Gain/1
  Constant/1 -> Divide/1
  pwr_dis_bat/1 -> Divide/2
  Gain/1 -> Divide/3
  mot_map3/1 -> MinMax3/1
  TrqLimU_dig_rr/1 -> MinMax3/2
  mot_map2/1 -> MinMax4/1
  TrqLimU_dig_rf/1 -> MinMax4/2
  mot_map1/1 -> MinMax5/1
  TrqLimU_dig_lr/1 -> MinMax5/2
  mot_map/1 -> MinMax6/1
  TrqLimU_dig_lf/1 -> MinMax6/2
  MinMax6/1 -> trqlim_lf/1, Add3/1
  MinMax5/1 -> trqlim_lr/1, Add3/2
  MinMax4/1 -> trqlim_rf/1, Add3/3
  MinMax3/1 -> trqlim_rr/1, Add3/4
  Divide/1 -> MinMax/1
  Add3/1 -> MinMax/2
  MinMax/1 -> Product/2
  acc_dem/1 -> Product/1
  Product/1 -> Gain1/1
  Gain1/1 -> trq_dem_r/1, trq_dem_l/1

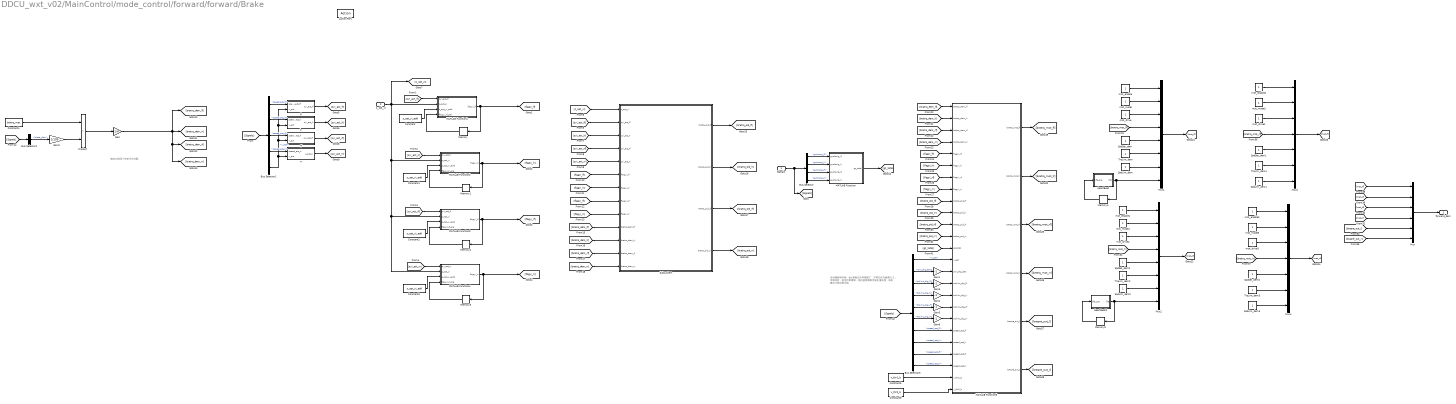
== system DDCU_wxt_v02/MainControl/mode_control/forward/forward/Brake ==
  note: 当时编程序时候，fcn里面正负号搞错了，不得已在外面乘以-1，
      | 当制动时，电池功率限制，电机扭矩限制当做正值处理，电机
      | 输出力矩也是正值
  note: 制动力矩四个车轮平均分配
  Signals : Inport
  s_opt_yi : Inport  Port=2
  Action Port : ActionPort  ActionType=case
  Bus Selector : BusSelector  OutputSignals=DriveMotor.guzhang_lf,DriveMotor.guzhang_lr,DriveMotor.guzhang_rf,DriveMotor.guzhang_rr
  Bus Selector1 : BusSelector  OutputSignals=DriveMotor.speed_act_lf,DriveMotor.speed_act_lr,DriveMotor.speed_act_rf,DriveMotor.speed_act_rr,IMU.v_act
  Bus Selector2 : BusSelector  OutputSignals=YaoKong.brake_dem
  Bus Selector3 : BusSelector  OutputSignals=IMU.v_act,Bat.pwr_chg_bat,DriveMotor.trqlimL_dig_lf,DriveMotor.trqlimL_dig_lr,DriveMotor.trqlimL_dig_rf,DriveMotor.trqlimL_dig_rr,DriveMotor.speed_act_lf,DriveMotor.speed_act_lr,DriveMotor.speed_act_rf,DriveMotor.speed_act_rr
  Constant{,1..3} (4 alike) : Constant  Value=s_opt_yi_add
  Constant4 : Constant  Value=bratrq_max
  Constant5 : Constant  Value=v_thr1_b
  Constant6 : Constant  Value=v_thr2_b
  Gain : Gain  Gain=1/4
  Gain{1,3..6} (5 alike) : Gain  Gain=-1
  Gain2 : Gain  Gain=1/100
  HeartBeat : MATLAB Function  TreatAsAtomicUnit=on
  HeartBeat1 : MATLAB Function  TreatAsAtomicUnit=on
  MATLAB Function : MATLAB Function  TreatAsAtomicUnit=on
  MATLAB Function1 : MATLAB Function  TreatAsAtomicUnit=on
  MATLAB Function2 : MATLAB Function  TreatAsAtomicUnit=on
  MATLAB Function3 : MATLAB Function  TreatAsAtomicUnit=on
  MATLAB Function4 : MATLAB Function  TreatAsAtomicUnit=on
  MATLAB Function5 : MATLAB Function  TreatAsAtomicUnit=on
  Memory{,1..5} (6 alike) : Memory
  Mux : Mux  Inputs=6
  Mux1 : Mux  Inputs=8
  Mux2 : Mux  Inputs=8
  Mux3 : Mux  Inputs=7
  Mux4 : Mux  Inputs=7
  Product : Product
  SpdLim_dem{,1..3} (4 alike) : Constant
  SpdSet_dem{,1..3} (4 alike) : Constant
  Subsystem : Subsystem
  TrqLim_dem{,1..3} (4 alike) : Constant
  lf : Subsystem
  lr : Subsystem
  mot_drive{,1..3} (4 alike) : Constant
  mot_enable{,1..3} (4 alike) : Constant
  mot_mode{,1..3} (4 alike) : Constant
  rf : Subsystem
  rr : Subsystem
  forward_dem : Outport
  wires:
  Signals/1 -> [Signals], Bus Selector/1
  Bus Selector/3 -> MATLAB Function/3(guzhang_rf)  "<guzhang_rf>"
  Bus Selector/4 -> MATLAB Function/4(guzhang_rr)  "<guzhang_rr>"
  Bus Selector/2 -> MATLAB Function/2(guzhang_lr)  "<guzhang_lr>"
  Bus Selector/1 -> MATLAB Function/1(guzhang_lf)  "<guzhang_lf>"
  MATLAB Function/1(gz_total) -> [gz_total]
  [Signals] -> Bus Selector1/1
  Bus Selector1/1 -> lf/1(speed_act_lf)  "<speed_act_lf>"
  Bus Selector1/2 -> lr/1(speed_act_lr)  "<speed_act_lr>"
  Bus Selector1/3 -> rf/1(speed_act_rf)  "<speed_act_rf>"
  Bus Selector1/4 -> rr/1(speed_act_rr)  "<speed_act_rr>"
  Bus Selector1/5 -> rr/2(v_act), rf/2(v_act), lr/2(v_act), lf/2(v_act)  "<v_act>"
  Constant3/1 -> MATLAB Function4/3(s_opt_yi_add)
  Memory3/1 -> MATLAB Function4/4(flagyi_rr_pre)
  MATLAB Function4/1(flagyi_rr) -> Memory3/1, [flagyi_rr]
  s_opt_yi/1 -> MATLAB Function2/2(s_opt_yi), MATLAB Function3/2(s_opt_yi), MATLAB Function4/2(s_opt_yi), MATLAB Function1/2(s_opt_yi), [s_opt_yi]
  Constant2/1 -> MATLAB Function3/3(s_opt_yi_add)
  Memory2/1 -> MATLAB Function3/4(flagyi_rf_pre)
  MATLAB Function3/1(flagyi_rf) -> [flagyi_rf], Memory2/1
  Constant1/1 -> MATLAB Function2/3(s_opt_yi_add)
  Memory1/1 -> MATLAB Function2/4(flagyi_lr_pre)
  MATLAB Function2/1(flagyi_lr) -> Memory1/1, [flagyi_lr]
  Constant/1 -> MATLAB Function1/3(s_opt_yi_add)
  Memory/1 -> MATLAB Function1/4(flagyi_lf_pre)
  MATLAB Function1/1(flagyi_lf) -> [flagyi_lf], Memory/1
  lr/1(syi_act_lr) -> [syi_act_lr]
  lf/1(syi_act_lf) -> [syi_act_lf]
  rf/1(syi_act_rf) -> [syi_act_rf]
  rr/1(s_act_rr) -> [syi_act_rr]
  [syi_act_lf] -> MATLAB Function1/1(syi_act_lf)
  [syi_act_lr] -> MATLAB Function2/1(syi_act_lr)
  [syi_act_rf] -> MATLAB Function3/1(syi_act_rf)
  [syi_act_rr] -> MATLAB Function4/1(syi_act_rr)
  [s_opt_yi] -> Subsystem/1(s_opt_yi)
  [syi_act_lf] -> Subsystem/2(syi_act_lf)
  [syi_act_lr] -> Subsystem/3(syi_act_lr)
  [syi_act_rf] -> Subsystem/4(syi_act_rf)
  [syi_act_rr] -> Subsystem/5(syi_act_rr)
  [flagyi_rf] -> Subsystem/8(flagyi_rf)
  [flagyi_lf] -> Subsystem/6(flagyi_lf)
  [flagyi_lr] -> Subsystem/7(flagyi_lr)
  [flagyi_rr] -> Subsystem/9(flagyi_rr)
  [Signals] -> Bus Selector2/1
  Gain/1 -> [bratrq_dem_lr], [bratrq_dem_rr], [bratrq_dem_rf], [bratrq_dem_lf]
  [bratrq_dem_lf] -> Subsystem/10(bratrq_dem_lf)
  [bratrq_dem_lr] -> Subsystem/11(bratrq_dem_lr)
  [bratrq_dem_rf] -> Subsystem/12(bratrq_dem_rf)
  [bratrq_dem_rr] -> Subsystem/13(bratrq_dem_rr)
  Subsystem/2(bratrq_pid_lr) -> [bratrq_pid_lr]
  Subsystem/3(bratrq_pid_rf) -> [bratrq_pid_rf]
  Subsystem/1(bratrq_pid_lf) -> [bratrq_pid_lf]
  Subsystem/4(bratrq_pid_rr) -> [bratrq_pid_rr]
  [bratrq_dem_rf] -> MATLAB Function5/3(bratrq_dem_rf)
  [bratrq_dem_lf] -> MATLAB Function5/1(bratrq_dem_lf)
  [bratrq_dem_lr] -> MATLAB Function5/2(bratrq_dem_lr)
  [bratrq_dem_rr] -> MATLAB Function5/4(bratrq_dem_rr)
  [flagyi_lf] -> MATLAB Function5/5(flagyi_lf)
  [flagyi_lr] -> MATLAB Function5/6(flagyi_lr)
  [flagyi_rf] -> MATLAB Function5/7(flagyi_rf)
  [flagyi_rr] -> MATLAB Function5/8(flagyi_rr)
  [bratrq_pid_rf] -> MATLAB Function5/11(bratrq_pid_rf)
  [bratrq_pid_rr] -> MATLAB Function5/12(bratrq_pid_rr)
  [bratrq_pid_lf] -> MATLAB Function5/9(bratrq_pid_lf)
  Mux/1 -> forward_dem/1
  SpdLim_dem3/1 -> Mux4/7
  TrqLim_dem3/1 -> Mux4/6
  Mux4/1 -> [mot_rr]
  SpdSet_dem3/1 -> Mux4/5
  mot_enable3/1 -> Mux4/1
  [bratrq_mot_rr] -> Mux4/4
  mot_mode3/1 -> Mux4/2
  mot_drive3/1 -> Mux4/3
  SpdLim_dem2/1 -> Mux2/7
  Memory5/1 -> HeartBeat1/1(life_pre)
  HeartBeat1/1(life) -> Memory5/1, Mux2/8
  TrqLim_dem2/1 -> Mux2/6
  Mux2/1 -> [mot_lr]
  SpdSet_dem2/1 -> Mux2/5
  mot_enable1/1 -> Mux2/1
  [bratrq_mot_lr] -> Mux2/4
  mot_mode1/1 -> Mux2/2
  mot_drive2/1 -> Mux2/3
  SpdLim_dem1/1 -> Mux3/7
  TrqLim_dem1/1 -> Mux3/6
  Mux3/1 -> [mot_rf]
  SpdSet_dem1/1 -> Mux3/5
  mot_enable2/1 -> Mux3/1
  [bratrq_mot_rf] -> Mux3/4
  mot_mode2/1 -> Mux3/2
  mot_drive1/1 -> Mux3/3
  SpdLim_dem/1 -> Mux1/7
  Memory4/1 -> HeartBeat/1(life_pre)
  HeartBeat/1(life) -> Memory4/1, Mux1/8
  TrqLim_dem/1 -> Mux1/6
  Mux1/1 -> [mot_lf]
  SpdSet_dem/1 -> Mux1/5
  mot_enable/1 -> Mux1/1
  [bratrq_mot_lf] -> Mux1/4
  mot_mode/1 -> Mux1/2
  mot_drive/1 -> Mux1/3
  [mot_lf] -> Mux/1
  [mot_lr] -> Mux/2
  [mot_rf] -> Mux/3
  [mot_rr] -> Mux/4
  [brapre_out_l] -> Mux/5
  [brapre_out_r] -> Mux/6
  MATLAB Function5/1(bratrq_mot_lf) -> [bratrq_mot_lf]
  MATLAB Function5/3(bratrq_mot_rf) -> [bratrq_mot_rf]
  MATLAB Function5/2(bratrq_mot_lr) -> [bratrq_mot_lr]
  MATLAB Function5/4(bratrq_mot_rr) -> [bratrq_mot_rr]
  MATLAB Function5/5(brapre_out_l) -> [brapre_out_l]
  MATLAB Function5/6(brapre_out_r) -> [brapre_out_r]
  [gz_total] -> MATLAB Function5/13(gz_total)
  [Signals] -> Bus Selector3/1
  Bus Selector3/2 -> Gain1/1  "<pwr_chg_bat>"
  Bus Selector3/1 -> MATLAB Function5/14(v_act)  "<v_act>"
  [bratrq_pid_lr] -> MATLAB Function5/10(bratrq_pid_lr)
  Bus Selector3/3 -> Gain3/1  "<trqlimL_dig_lf>"
  Bus Selector3/4 -> Gain4/1  "<trqlimL_dig_lr>"
  Bus Selector3/5 -> Gain5/1  "<trqlimL_dig_rf>"
  Bus Selector3/6 -> Gain6/1  "<trqlimL_dig_rr>"
  Bus Selector3/7 -> MATLAB Function5/20(speed_act_lf)  "<speed_act_lf>"
  Bus Selector3/8 -> MATLAB Function5/21(speed_act_lr)  "<speed_act_lr>"
  Bus Selector3/9 -> MATLAB Function5/22(speed_act_rf)  "<speed_act_rf>"
  Bus Selector3/10 -> MATLAB Function5/23(speed_act_rr)  "<speed_act_rr>"
  Constant4/1 -> Product/1
  Gain2/1 -> Product/2
  Bus Selector2/1 -> Gain2/1  "<brake_dem>"
  Product/1 -> Gain/1
  Constant5/1 -> MATLAB Function5/24(v_thr1_b)
  Constant6/1 -> MATLAB Function5/25(v_thr2_b)
  Gain1/1 -> MATLAB Function5/15(pwr_chg_bat)
  Gain3/1 -> MATLAB Function5/16(trqlimL_dig_lf)
  Gain4/1 -> MATLAB Function5/17(trqlimL_dig_lr)
  Gain5/1 -> MATLAB Function5/18(trqlimL_dig_rf)
  Gain6/1 -> MATLAB Function5/19(trqlimL_dig_rr)

== system DDCU_wxt_v02/MainControl/mode_control/forward/forward/Drive ==
  Signals : Inport
  Action Port : ActionPort  ActionType=case
  Bus Selector : BusSelector  OutputSignals=YaoKong.acc_dem,IMU.v_act,DriveMotor.trqlimU_dig_lf,DriveMotor.trqlimU_dig_lr,DriveMotor.trqlimU_dig_rf,DriveMotor.trqlimU_dig_rr
  Bus Selector1 : BusSelector  OutputSignals=IMU.acc_y
  Bus Selector2 : BusSelector  OutputSignals=IMU.acc_y,YaoKong.steer_dem
  Bus Selector3 : BusSelector  OutputSignals=IMU.dis_east,IMU.dis_north,IMU.hangxiangangle
  Bus Selector4 : BusSelector  OutputSignals=IMU.v_act,DriveMotor.trqlimU_dig_lf,DriveMotor.trqlimU_dig_lr,DriveMotor.trqlimU_dig_rf,DriveMotor.trqlimU_dig_rr,YaoKong.steer_dem
  Bus Selector5 : BusSelector  OutputSignals=Bat.pwr_dis_bat,DriveMotor.speed_act_lf,DriveMotor.speed_act_lr,DriveMotor.speed_act_rf,DriveMotor.speed_act_rr,DriveMotor.trqlimU_dig_lf,DriveMotor.trqlimU_dig_lr,DriveMotor.trqlimU_dig_rf,DriveMotor.trqlimU_dig_rr
  Bus Selector6 : BusSelector  OutputSignals=DriveMotor.guzhang_lf,DriveMotor.guzhang_lr,DriveMotor.guzhang_rf,DriveMotor.guzhang_rr
  Bus Selector7 : BusSelector  OutputSignals=DriveMotor.speed_act_lf,DriveMotor.speed_act_lr,DriveMotor.speed_act_rf,DriveMotor.speed_act_rr,IMU.v_act,YaoKong.steer_dem,IMU.acc_y,YaoKong.brake_dem
  Constant : Constant  Value=ag_thr
  Constant1 : Constant
  MATLAB Function : MATLAB Function  TreatAsAtomicUnit=on
  Multiport Switch : MultiPortSwitch  DataPortOrder=Zero-based contiguous
  Switch Case : SwitchCase  CaseConditions={0,1,2}  ShowDefaultCase=off
  Terminator : Terminator
  容错控制 : Subsystem
  左右侧电机分配及功率限制 : Subsystem
  目标直驶力矩确定模块 : Subsystem
  目标转向力矩确定模块 : Subsystem  TreatAsAtomicUnit=on
  直驶纠偏控制 : Subsystem  TreatAsAtomicUnit=on
  路面状况识别模块 : Subsystem
  车辆稳定性控制 : Subsystem  TreatAsAtomicUnit=on
  驱动防滑控制TCS : Subsystem
  forward_dem : Outport
  wires:
  Signals/1 -> [Signals], Bus Selector4/1, Bus Selector3/1, Bus Selector1/1, Bus Selector2/1, Bus Selector/1
  Bus Selector/1 -> 目标直驶力矩确定模块/1(acc_dem)  "<acc_dem>"
  Bus Selector/2 -> 目标直驶力矩确定模块/2(v_act)  "<v_act>"
  Bus Selector1/1 -> 车辆稳定性控制/1(acc_y)  "<acc_y>"
  MATLAB Function/1(y) -> Multiport Switch/1, Switch Case/1
  Switch Case/1 -> 车辆稳定性控制/Action
  Switch Case/2 -> 目标转向力矩确定模块/Action
  Switch Case/3 -> 直驶纠偏控制/Action
  车辆稳定性控制/1(delta_Twending_dem) -> Multiport Switch/2
  目标转向力矩确定模块/1(delta_Tsteer_dem) -> Multiport Switch/3
  直驶纠偏控制/1(delta_Tjiupian) -> Multiport Switch/4
  Bus Selector2/2 -> MATLAB Function/2(steer_dem)  "<steer_dem>"
  Constant/1 -> MATLAB Function/3(ag_thr)
  [umax] -> 目标转向力矩确定模块/7(umax)
  [f] -> 目标转向力矩确定模块/8(f)
  路面状况识别模块/1(umax) -> [umax]
  路面状况识别模块/2(f) -> [f]
  路面状况识别模块/3(s_opt_zhuan) -> [s_opt_zhuan]
  Bus Selector3/1 -> 直驶纠偏控制/1(dis_east)  "<dis_east>"
  Bus Selector3/2 -> 直驶纠偏控制/2(dis_north)  "<dis_north>"
  Bus Selector3/3 -> 直驶纠偏控制/3(hangxiangangle)  "<hangxiangangle>"
  Multiport Switch/1 -> 左右侧电机分配及功率限制/2(delta_T_dem)
  目标直驶力矩确定模块/1(Trq_line_dem) -> 左右侧电机分配及功率限制/1(Trq_line_dem)
  Bus Selector/4 -> 目标直驶力矩确定模块/4(TrqLimU_dig_lr)  "<trqlimU_dig_lr>"
  Bus Selector/3 -> 目标直驶力矩确定模块/3(TrqLimU_dig_lf)  "<trqlimU_dig_lf>"
  Bus Selector/5 -> 目标直驶力矩确定模块/5(TrqLimU_dig_rf)  "<trqlimU_dig_rf>"
  Bus Selector/6 -> 目标直驶力矩确定模块/6(TrqLimU_dig_rr)  "<trqlimU_dig_rr>"
  Bus Selector4/4 -> 目标转向力矩确定模块/4(TrqLimU_dig_rf)  "<trqlimU_dig_rf>"
  Bus Selector4/5 -> 目标转向力矩确定模块/5(TrqLimU_dig_rr)  "<trqlimU_dig_rr>"
  Bus Selector4/6 -> 目标转向力矩确定模块/6(steer_dem)  "<steer_dem>"
  Bus Selector4/1 -> 目标转向力矩确定模块/1(v_act)  "<v_act>"
  Bus Selector4/2 -> 目标转向力矩确定模块/2(TrqLimU_dig_lf)  "<trqlimU_dig_lf>"
  Bus Selector4/3 -> 目标转向力矩确定模块/3(TrqLimU_dig_lr)  "<trqlimU_dig_lr>"
  Bus Selector2/1 -> MATLAB Function/1(acc_y)  "<acc_y>"
  [Signals] -> Bus Selector5/1
  Bus Selector5/1 -> 左右侧电机分配及功率限制/3(pwr_dis_bat)  "<pwr_dis_bat>"
  Bus Selector5/2 -> 左右侧电机分配及功率限制/4(speed_act_lf)  "<speed_act_lf>"
  Bus Selector5/3 -> 左右侧电机分配及功率限制/5(speed_act_lr)  "<speed_act_lr>"
  Bus Selector5/4 -> 左右侧电机分配及功率限制/6(speed_act_rf)  "<speed_act_rf>"
  Bus Selector5/5 -> 左右侧电机分配及功率限制/7(speed_act_rr)  "<speed_act_rr>"
  Bus Selector5/9 -> 左右侧电机分配及功率限制/11(TrqLimU_dig_rr)  "<trqlimU_dig_rr>"
  Bus Selector5/8 -> 左右侧电机分配及功率限制/10(TrqLimU_dig_rf)  "<trqlimU_dig_rf>"
  Bus Selector5/6 -> 左右侧电机分配及功率限制/8(TrqLimU_dig_lf)  "<trqlimU_dig_lf>"
  Bus Selector5/7 -> 左右侧电机分配及功率限制/9(TrqLimU_dig_lr)  "<trqlimU_dig_lr>"
  [Signals] -> Bus Selector6/1
  左右侧电机分配及功率限制/2(trq_dem_r) -> 容错控制/2(trq_dem_r)
  左右侧电机分配及功率限制/1(trq_dem_l) -> 容错控制/1(trq_dem_l)
  Bus Selector6/4 -> 容错控制/10(guzhang_rr)  "<guzhang_rr>"
  Bus Selector6/3 -> 容错控制/9(guzhang_rf)  "<guzhang_rf>"
  Bus Selector6/2 -> 容错控制/8(guzhang_lr)  "<guzhang_lr>"
  Bus Selector6/1 -> 容错控制/7(guzhang_lf)  "<guzhang_lf>"
  左右侧电机分配及功率限制/5(trqlim_rf) -> 容错控制/5(trqlim_rf)
  左右侧电机分配及功率限制/4(trqlim_lr) -> 容错控制/4(trqlim_lr)
  左右侧电机分配及功率限制/6(trqlim_rr) -> 容错控制/6(trqlim_rr)
  左右侧电机分配及功率限制/3(trqlim_lf) -> 容错控制/3(trqlim_lf)
  容错控制/1(trq_dem_lf) -> 驱动防滑控制TCS/1(trq_dem_lf)
  容错控制/5(bra_pre_l) -> 驱动防滑控制TCS/5(bra_pre_l)
  容错控制/6(bra_pre_r) -> 驱动防滑控制TCS/6(bra_pre_r)
  容错控制/2(trq_dem_lr) -> 驱动防滑控制TCS/2(trq_dem_lr)
  容错控制/3(trq_dem_rf) -> 驱动防滑控制TCS/3(trq_dem_rf)
  容错控制/4(trq_dem_rr) -> 驱动防滑控制TCS/4(trq_dem_rr)
  Bus Selector7/7 -> 驱动防滑控制TCS/13(acc_y)  "<acc_y>"
  Bus Selector7/6 -> 驱动防滑控制TCS/12(steer_dem)  "<steer_dem>"
  Bus Selector7/5 -> 驱动防滑控制TCS/11(v_act)  "<v_act>"
  Bus Selector7/4 -> 驱动防滑控制TCS/10(speed_act_rr)  "<speed_act_rr>"
  Bus Selector7/3 -> 驱动防滑控制TCS/9(speed_act_rf)  "<speed_act_rf>"
  Bus Selector7/2 -> 驱动防滑控制TCS/8(speed_act_lr)  "<speed_act_lr>"
  Bus Selector7/1 -> 驱动防滑控制TCS/7(speed_act_lf)  "<speed_act_lf>"
  [s_opt_zhuan] -> 驱动防滑控制TCS/15(s_opt_zhuan)
  Bus Selector7/8 -> 驱动防滑控制TCS/14(brake_dem)  "<brake_dem>"
  [Signals] -> Bus Selector7/1
  驱动防滑控制TCS/1(forward_dem) -> forward_dem/1
  Constant1/1 -> 路面状况识别模块/1(In1)
  路面状况识别模块/4(s_opt_yi) -> Terminator/1

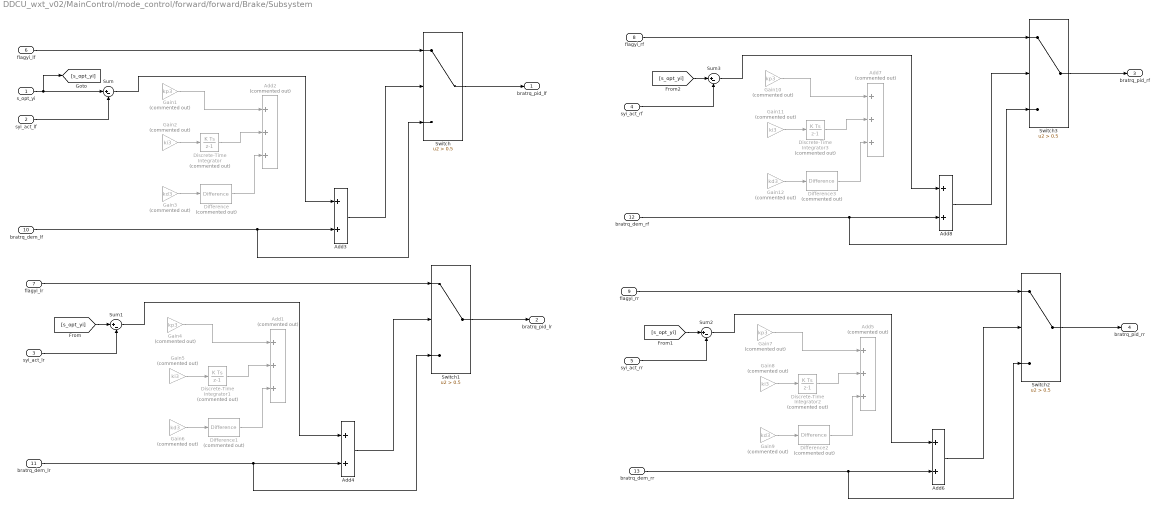
== system DDCU_wxt_v02/MainControl/mode_control/forward/forward/Brake/Subsystem ==
  s_opt_yi : Inport
  syi_act_lf : Inport  Port=2
  syi_act_lr : Inport  Port=3
  syi_act_rf : Inport  Port=4
  syi_act_rr : Inport  Port=5
  flagyi_lf : Inport  Port=6
  flagyi_lr : Inport  Port=7
  flagyi_rf : Inport  Port=8
  flagyi_rr : Inport  Port=9
  bratrq_dem_lf : Inport  Port=10
  bratrq_dem_lr : Inport  Port=11
  bratrq_dem_rf : Inport  Port=12
  bratrq_dem_rr : Inport  Port=13
  Add{1..2,5,7} (4 alike) : Sum  Commented=on  Inputs=+++
  Add{3..4,6,8} (4 alike) : Sum
  Difference{,1..3} (4 alike) : simulink/Discrete/Difference  Commented=on  ICPrevInput=0.0  InputProcessing=Inherited  OutMin=[]  OutMax=[]  OutDataType=fixdt(1, 16)  OutScaling=2^-10  DoSatur=off
  Discrete-Time Integrator{,1..3} (4 alike) : DiscreteIntegrator  Commented=on  SampleTime=-1  ICPrevOutput=DiscIntNeverNeededParam  ICPrevScaledInput=DiscIntNeverNeededParam
  Gain{1,4,7,10} (4 alike) : Gain  Commented=on  Gain=kp3
  Gain{2,5,8,11} (4 alike) : Gain  Commented=on  Gain=ki3
  Gain{3,6,9,12} (4 alike) : Gain  Commented=on  Gain=kd3
  Sum{,1..3} (4 alike) : Sum  Inputs=|+-
  Switch{,1..3} (4 alike) : Switch  Criteria=u2 > Threshold  Threshold=0.5
  bratrq_pid_lf : Outport
  bratrq_pid_lr : Outport  Port=2
  bratrq_pid_rf : Outport  Port=3
  bratrq_pid_rr : Outport  Port=4
  wires:
  Add3/1 -> Switch/2
  bratrq_dem_lf/1 -> Switch/3, Add3/2
  syi_act_lf/1 -> Sum/2
  Difference/1 -> Add2/3
  Discrete-Time Integrator/1 -> Add2/2
  Gain3/1 -> Difference/1
  Gain1/1 -> Add2/1
  Gain2/1 -> Discrete-Time Integrator/1
  s_opt_yi/1 -> [s_opt_yi], Sum/1
  flagyi_lf/1 -> Switch/1
  Switch/1 -> bratrq_pid_lf/1
  Add4/1 -> Switch1/2
  bratrq_dem_lr/1 -> Switch1/3, Add4/2
  syi_act_lr/1 -> Sum1/2
  Difference1/1 -> Add1/3
  Discrete-Time Integrator1/1 -> Add1/2
  Gain6/1 -> Difference1/1
  Gain4/1 -> Add1/1
  Gain5/1 -> Discrete-Time Integrator1/1
  [s_opt_yi] -> Sum1/1
  flagyi_lr/1 -> Switch1/1
  Switch1/1 -> bratrq_pid_lr/1
  Add6/1 -> Switch2/2
  bratrq_dem_rr/1 -> Switch2/3, Add6/2
  syi_act_rr/1 -> Sum2/2
  Difference2/1 -> Add5/3
  Discrete-Time Integrator2/1 -> Add5/2
  Gain9/1 -> Difference2/1
  Gain7/1 -> Add5/1
  Gain8/1 -> Discrete-Time Integrator2/1
  [s_opt_yi] -> Sum2/1
  flagyi_rr/1 -> Switch2/1
  Switch2/1 -> bratrq_pid_rr/1
  Add8/1 -> Switch3/2
  bratrq_dem_rf/1 -> Switch3/3, Add8/2
  syi_act_rf/1 -> Sum3/2
  Difference3/1 -> Add7/3
  Discrete-Time Integrator3/1 -> Add7/2
  Gain12/1 -> Difference3/1
  Gain10/1 -> Add7/1
  Gain11/1 -> Discrete-Time Integrator3/1
  [s_opt_yi] -> Sum3/1
  flagyi_rf/1 -> Switch3/1
  Switch3/1 -> bratrq_pid_rf/1
  Sum/1 -> Add3/1
  Sum1/1 -> Add4/1
  Sum3/1 -> Add8/1
  Sum2/1 -> Add6/1

== system DDCU_wxt_v02/MainControl/mode_control/forward/forward/Brake/lf ==
  speed_act_lf : Inport
  v_act : Inport  Port=2
  Add : Sum
  Constant : Constant  Value=eps
  Divide : Product  Inputs=*/
  Gain : Gain  Gain=pi/30
  Gain1 : Gain  Gain=Radius
  Gain2 : Gain  Gain=1/3.6
  Subtract : Sum  Inputs=+-
  syi_act_lf : Outport
  wires:
  Divide/1 -> syi_act_lf/1
  Add/1 -> Divide/2
  Constant/1 -> Add/2
  Subtract/1 -> Divide/1
  v_act/1 -> Gain2/1
  Gain/1 -> Gain1/1
  speed_act_lf/1 -> Gain/1
  Gain2/1 -> Add/1, Subtract/1
  Gain1/1 -> Subtract/2
